simulink model "Exercitiul5"  (R2016a)
settings: Solver=VariableStepDiscrete  StartTime=0.0  StopTime=2400  RelTol=1e-3
undefined symbols (not defined in the file): m, n
settings Model: Creator=Cristina  LastModifiedBy=Cristina

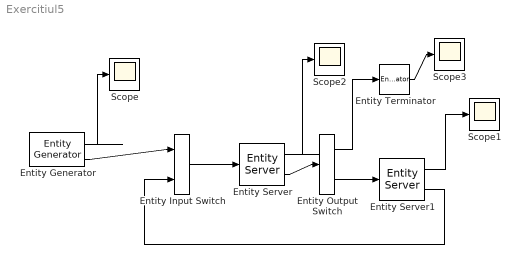
== system Exercitiul5 ==
  Entity Input Switch : EntityInputSwitch  InputPortMessageModes=m,m  OutputPortMessageModes=m
  Entity Output Switch : EntityOutputSwitch  InputPortMessageModes=m  OutputPortMessageModes=m,m  SwitchingCriterion=From attribute  SwitchAttributeName=priority
  Entity Generator : EntityGenerator  OutputPortMessageModes=n,m  AttributeName=priority  AttributeInitialValue=2  NumberEntitiesDeparted=on  EntityType=Structured  EntityTypeName=Entity
      settings: OutputPortMap=o0,o3
  Entity Server : EntityServer  InputPortMessageModes=m  OutputPortMessageModes=n,m  Capacity=4  ServiceTimeSource=MATLAB action  ServiceTimeAction=dt = 10 * rand + 25;  NumberEntitiesDeparted=on
      settings: OutputPortMap=o0,o9
  Entity Server1 : EntityServer  InputPortMessageModes=m  OutputPortMessageModes=n,m  Capacity=1  ServiceTimeSource=MATLAB action  ServiceTimeAction=dt = 4 * rand + 6;  EntryAction=entity.priority = 1;  NumberEntitiesDeparted=on
      settings: OutputPortMap=o0,o9
  Entity Terminator : EntityTerminator  InputPortMessageModes=m  NumberEntitiesArrived=on
      settings: OutputPortMap=o0
  Scope{,1..3} (4 alike) : Scope
  wires:
  Entity Server1/2 -> Entity Input Switch/2
  Entity Generator/2 -> Entity Input Switch/1
  Entity Input Switch/1 -> Entity Server/1
  Entity Generator/1 -> Scope/1
  Entity Server/1 -> Scope2/1
  Entity Server1/1 -> Scope1/1
  Entity Server/2 -> Entity Output Switch/1
  Entity Output Switch/2 -> Entity Server1/1
  Entity Output Switch/1 -> Entity Terminator/1
  Entity Terminator/1 -> Scope3/1
